simulink model "roomtemp7"  (R2017b)
settings: Solver=ode45  StartTime=0.0  StopTime=86400  MaxStep=10  MinStep=0.00000001  RelTol=1e-6  AbsTol=1e-6  EnableMultiTasking=on
undefined symbols (not defined in the file or in its folder): C1, Cf, Ch, Cw1, Cw2, Cwi, Cwo, Fii_i1, R1, Rc1, Rc2, Rc3, Rext, Rf1, Rf2, Rground, Rheater, Rw
libraries: simulink x4, dsparch4 x1
settings Model: Creator=Andres  LastModifiedBy=Andres
settings DataIOCC: LimitDataPoints=on  SaveFormat=Array  SignalLoggingSaveFormat=ModelDataLogs  SaveOutput=off  SaveTime=off  SignalLoggingName=sigsOut
settings OptimizationCC: ExpressionDepthLimit=2147483647  InitFltsAndDblsToZero=on  LifeSpan=inf
settings DebuggingCC: SaveWithParameterizedLinksMsg=none  UnderspecifiedInitializationDetection=Classic  MergeDetectMultiDrivingBlocksExec=none  SignalResolutionControl=TryResolveAllWithWarning  MultiTaskDSMMsg=warning  MultiTaskCondExecSysMsg=none  FcnCallInpInsideContextMsg=warning  StateNameClashWarn=warning  StrictBusMsg=None  SFUnexpectedBacktrackingDiag=warning  SFNoUnconditionalDefaultTransitionDiag=warning  SFExecutionAtInitializationDiag=none
settings HardwareCC: ProdBitPerPointer=32  ProdBitPerSizeT=32  ProdBitPerPtrDiffT=32  ProdLargestAtomicFloat=None  ProdIntDivRoundTo=Undefined  ProdEndianess=Unspecified  ProdWordSize=32  ProdHWDeviceType=32-bit Generic  TargetUnknown=on
settings ModelReferenceCC: PropagateSignalLabelsOutOfModel=off
settings CodeAppCC: StateflowObjectComments=on
settings GRTTargetCC: TargetFcnLib=ansi_tfl_tmw.mat  TargetLangStandard=C89/C90 (ANSI)  CombineOutputUpdateFcns=off  GRTInterface=on
settings ConfigComp: CovMetricSettings=dw  CovHtmlReporting=on  CovSaveCumulativeToWorkspaceVar=on  CovSaveSingleToWorkspaceVar=on  CovExternalEMLEnable=off

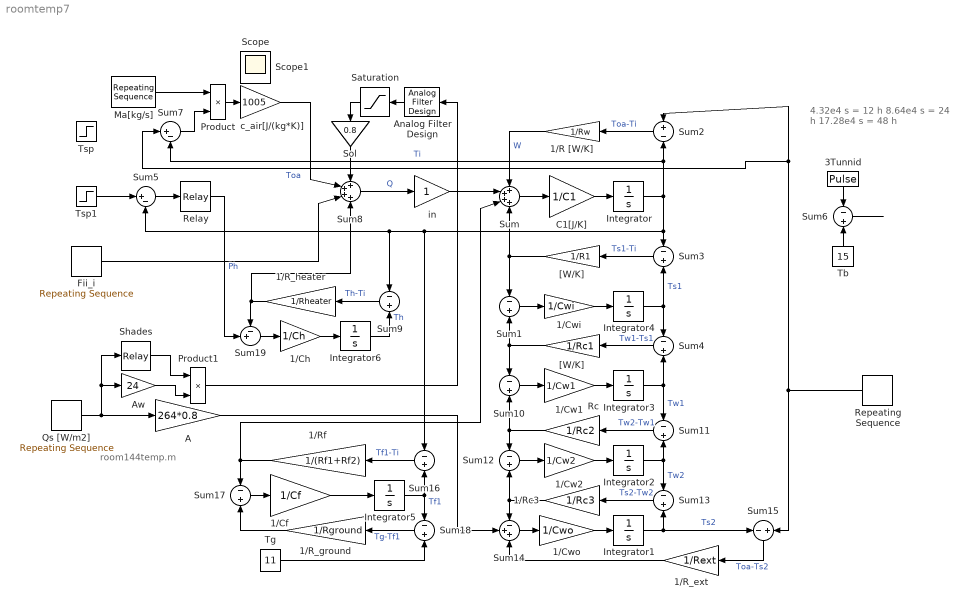
== system roomtemp7 ==
  note: room144temp.m
  note: 4.32e4 s = 12 h
      | 8.64e4 s = 24 h
      | 17.28e4 s = 48 h
  " 1/R_ext" : Gain  Gain=1/Rext
  " 1/R_ground" : Gain  Gain=1/Rground
  " 1/R_heater" : Gain  Gain=1/Rheater
  " 1/Rc3" : Gain  Gain=1/Rc3
  " 1/Rf" : Gain  Gain=1/(Rf1+Rf2)
  " Rc" : Gain  Gain=1/Rc2
  " [W/K]" : Gain  Gain=1/Rc1
  1/Cf : Gain  Gain=1/Cf
  1/Ch : Gain  Gain=1/Ch
  1/Cw1 : Gain  Gain=1/Cw1
  1/Cw2 : Gain  Gain=1/Cw2
  1/Cwi : Gain  Gain=1/Cwi
  1/Cwo : Gain  Gain=1/Cwo
  1/R [W/K] : Gain  Gain=1/Rw
  3Tunnid : DiscretePulseGenerator  PulseType=Time based  Amplitude=-1  Period=3600*3  PulseWidth=0.01
  A : Gain  Gain=264*0.8
  Analog Filter Design : dsparch4/Analog Filter Design  method=Butterworth  filttype=Lowpass  N=8  Wlo=0.0007  Whi=80  Rp=2  Rs=40
  Aw : Gain  Gain=24
  C1[J/K] : Gain  Gain=1/C1
  Fii_i : simulink/Sources/Repeating Sequence  rep_seq_t="[0  8.9 9 12 12.1 12.9 13 18  18.1 24]*3600"  rep_seq_y="[0  0    5  5   0      0   20     5   0    0]*Fii_i1"
  Integrator : Integrator  InitialCondition=15.5
  Integrator1 : Integrator  InitialCondition=11
  Integrator2 : Integrator  InitialCondition=12
  Integrator3 : Integrator  InitialCondition=13
  Integrator4 : Integrator  InitialCondition=15
  Integrator5 : Integrator  InitialCondition=12
  Integrator6 : Integrator  InitialCondition=15.5
  Ma[kg/s] : simulink/Sources/Repeating Sequence  rep_seq_t="[0  14.9 15    17  17.1  18 24] *3600"  rep_seq_y="[0    0    3.5  3.5   0     0    0 ]"
  Product : Product  RndMeth=Zero
  Product1 : Product  RndMeth=Zero
  Qs [W/m2] : simulink/Sources/Repeating Sequence  rep_seq_t="[0  8.4 8.5  9  10    11   12    15  16 17 17.3 24] *3600"  rep_seq_y="[0   0   65  70 100  250 180  100  80 75 0   0]"
  Relay : Relay  OnSwitchValue=0.5  OffSwitchValue=-0.5  OnOutputValue=8000
  Repeating Sequence : simulink/Sources/Repeating Sequence  rep_seq_t="[0    1     7    8   13  15   16 21 24] *3600"  rep_seq_y="[11 10.5 10 10.5 15 15.4  15  12 11]"
  Saturation : Saturate  UpperLimit=4000  LowerLimit=0
  Shades : Relay  OnSwitchValue=150  OffSwitchValue=130  OnOutputValue=0  OffOutputValue=1
  Sol : Gain  Gain=0.8
  Sum : Sum  Inputs=++++
  Sum{1,3..4,6,9..13,15..18} (13 alike) : Sum  Inputs=-+
  Sum14 : Sum  Inputs=-++
  Sum19 : Sum  Inputs=-+|
  Sum2 : Sum  Inputs=+-
  Sum5 : Sum  Inputs=|+-
  Sum7 : Sum  Inputs=|+-
  Sum8 : Sum  Inputs=++++
  Tb : Constant  Value=15
  Tg : Constant  Value=11
  Tsp : Step  Time=12*3600  Before=11  After=15  SampleTime=0
  Tsp1 : Step  Time=8*3600  After=0  SampleTime=0
  "[W/K]" : Gain  Gain=1/R1
  c_air[J/(kg*K)] : Gain  Gain=1005
  in : Gain
  Scope : Scope
  Scope1 : Scope
  wires:
  Integrator/1 -> Sum3/1, Sum16/1, Sum5/2, Sum9/1, Sum2/2, Sum7/2  "Ti"
  "[W/K]"/1 -> Sum/4, Sum1/1
  Sum1/1 -> 1/Cwi/1
  " [W/K]"/1 -> Sum10/1, Sum1/2
  Integrator4/1 -> Sum4/1, Sum3/2  "Ts1"
  1/R [W/K]/1 -> Sum/1  "W"
  C1[J/K]/1 -> Integrator/1
  1/Cwi/1 -> Integrator4/1
  Sum2/1 -> 1/R [W/K]/1  "Toa-Ti"
  Repeating Sequence/1 -> Sum15/2, Sum7/1, Sum2/1  "Toa"
  Sum3/1 -> "[W/K]"/1  "Ts1-Ti"
  Sum4/1 -> " [W/K]"/1  "Tw1-Ts1"
  Sum5/1 -> Relay/1
  Fii_i/1 -> Sum8/3
  Sum/1 -> C1[J/K]/1
  3Tunnid/1 -> Sum6/1
  Product/1 -> c_air[J/(kg*K)]/1
  Ma[kg/s]/1 -> Product/1
  Sum7/1 -> Product/2
  Sum8/1 -> in/1  "Q"
  in/1 -> Sum/2
  Tsp1/1 -> Sum5/1
  Integrator3/1 -> Sum11/1, Sum4/2  "Tw1"
  1/Cw1/1 -> Integrator3/1
  Sum10/1 -> 1/Cw1/1
  Integrator2/1 -> Sum13/1, Sum11/2  "Tw2"
  Sum11/1 -> " Rc"/1  "Tw2-Tw1"
  " Rc"/1 -> Sum12/1, Sum10/2
  1/Cw2/1 -> Integrator2/1
  Sum12/1 -> 1/Cw2/1
  Sum13/1 -> " 1/Rc3"/1  "Ts2-Tw2"
  " 1/Rc3"/1 -> Sum14/1, Sum12/2
  Integrator1/1 -> Sum15/1, Sum13/2  "Ts2"
  1/Cwo/1 -> Integrator1/1
  Sum14/1 -> 1/Cwo/1
  Sum15/1 -> " 1/R_ext"/1  "Toa-Ts2"
  " 1/R_ext"/1 -> Sum14/3
  Sum17/1 -> 1/Cf/1
  1/Cf/1 -> Integrator5/1
  Integrator5/1 -> Sum18/1, Sum16/2  "Tf1"
  " 1/Rf"/1 -> Sum17/1, Sum/3
  Sum16/1 -> " 1/Rf"/1  "Tf1-Ti"
  " 1/R_ground"/1 -> Sum17/2
  Tg/1 -> Sum18/2
  Sum18/1 -> " 1/R_ground"/1  "Tg-Tf1"
  Sum9/1 -> " 1/R_heater"/1  "Th-Ti"
  Integrator6/1 -> Sum9/2  "Th"
  " 1/R_heater"/1 -> Sum19/1, Sum8/4
  Sum19/1 -> 1/Ch/1
  1/Ch/1 -> Integrator6/1
  Relay/1 -> Sum19/2  "Ph"
  Tb/1 -> Sum6/2
  Sum6/1 -> ?
  Analog Filter Design/1 -> Saturation/1
  Sol/1 -> Sum8/1
  Saturation/1 -> Sol/1
  c_air[J/(kg*K)]/1 -> Sum8/2
  Qs [W/m2]/1 -> A/1, Shades/1, Aw/1
  Product1/1 -> Analog Filter Design/1
  A/1 -> Sum14/2
  Aw/1 -> Product1/2
  Shades/1 -> Product1/1
